simulink model "pm_and_pe_model"  (R2023a)
settings: Solver=VariableStepAuto  StartTime=0.0  StopTime=40*d  RelTol=1e-3
undefined symbols (not defined in the file): d
settings Model: Creator=enes  LastModifiedBy=enes

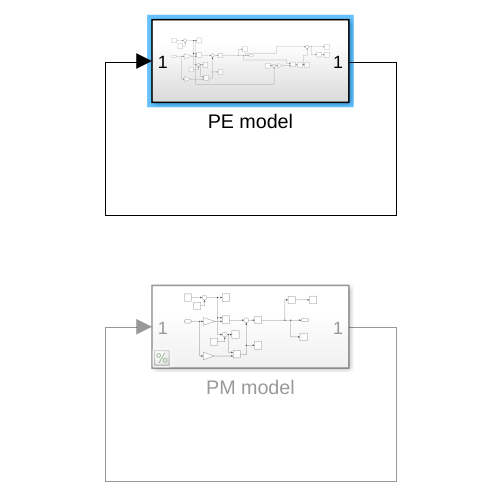
[thumbnail: Simulink's stored preview of the top-level diagram]
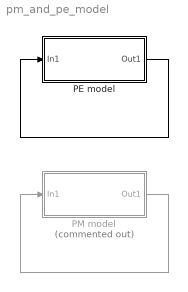
== system pm_and_pe_model ==
  PE model : Subsystem
  PM model : Subsystem  Commented=on
  wires:
  PE model/1(Out1) -> PE model/1(In1)
  PM model/1(Out1) -> PM model/1(In1)

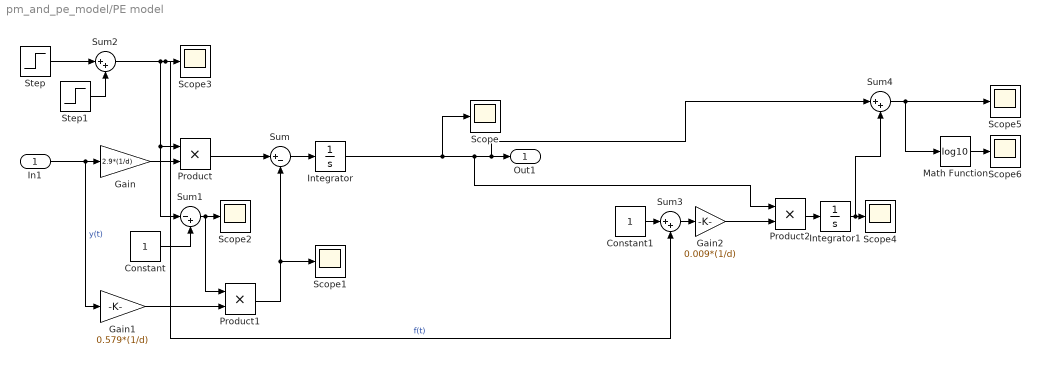
== system pm_and_pe_model/PE model ==
  In1 : Inport
  Constant : Constant
  Constant1 : Constant
  Gain : Gain  Gain=2.9*(1/d)
  Gain1 : Gain  Gain=0.579*(1/d)
  Gain2 : Gain  Gain=0.009*(1/d)
  Integrator : Integrator  InitialCondition=100
  Integrator1 : Integrator
  Math Function : Math  Operator=log10
  Product : Product
  Product1 : Product
  Product2 : Product
  Scope{,1..6} (7 alike) : Scope
  Step : Step  Time=5.9*d  Before=1  After=0  SampleTime=0
  Step1 : Step  Time=1.3*d  Before=-1  After=0  SampleTime=0
  Sum : Sum  Inputs=|+-
  Sum1 : Sum  Inputs=|-+
  Sum2 : Sum  Inputs=|++
  Sum3 : Sum  Inputs=|++
  Sum4 : Sum  Inputs=|++
  Out1 : Outport
  wires:
  Step1/1 -> Sum2/2
  Sum2/1 -> Sum3/2, Scope3/1, Sum1/1, Product/1  "f(t)"
  Step/1 -> Sum2/1
  In1/1 -> Gain1/1, Gain/1  "y(t)"
  Gain/1 -> Product/2
  Product/1 -> Sum/1
  Gain1/1 -> Product1/2
  Product1/1 -> Sum/2, Scope1/1
  Constant/1 -> Sum1/2
  Sum1/1 -> Product1/1, Scope2/1
  Sum/1 -> Integrator/1
  Integrator/1 -> Scope/1, Product2/1, Sum4/1, Out1/1
  Constant1/1 -> Sum3/1
  Sum3/1 -> Gain2/1
  Gain2/1 -> Product2/2
  Product2/1 -> Integrator1/1
  Integrator1/1 -> Sum4/2, Scope4/1
  Sum4/1 -> Math Function/1, Scope5/1
  Math Function/1 -> Scope6/1

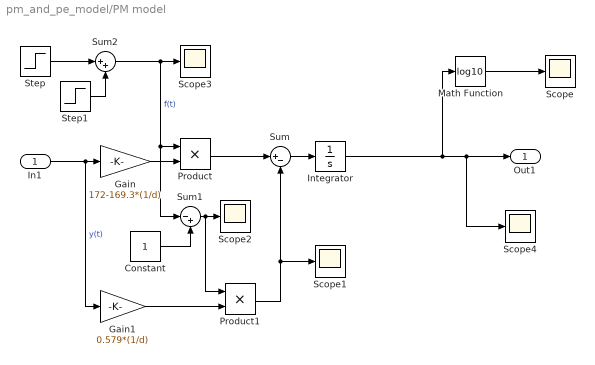
== system pm_and_pe_model/PM model ==
  In1 : Inport
  Constant : Constant
  Gain : Gain  Gain=172-169.3*(1/d)
  Gain1 : Gain  Gain=0.579*(1/d)
  Integrator : Integrator  InitialCondition=100
  Math Function : Math  Operator=log10
  Product : Product
  Product1 : Product
  Scope{,1..4} (5 alike) : Scope
  Step : Step  Time=5.98*d  Before=1  After=0  SampleTime=0
  Step1 : Step  Time=2.54*d  Before=-1  After=0  SampleTime=0
  Sum : Sum  Inputs=|+-
  Sum1 : Sum  Inputs=|-+
  Sum2 : Sum  Inputs=|++
  Out1 : Outport
  wires:
  Step1/1 -> Sum2/2
  Sum2/1 -> Scope3/1, Sum1/1, Product/1  "f(t)"
  Step/1 -> Sum2/1
  In1/1 -> Gain1/1, Gain/1  "y(t)"
  Gain/1 -> Product/2
  Product/1 -> Sum/1
  Gain1/1 -> Product1/2
  Product1/1 -> Sum/2, Scope1/1
  Constant/1 -> Sum1/2
  Sum1/1 -> Product1/1, Scope2/1
  Sum/1 -> Integrator/1
  Integrator/1 -> Math Function/1, Scope4/1, Out1/1
  Math Function/1 -> Scope/1
